simulink model "Pacejka_Tyre_Model"  (R2023b)
settings: Solver=VariableStepAuto  StartTime=0.0  StopTime=20  MinStep=1e-1  RelTol=1e-3
PostLoadFcn:
  | % loading model params:
  | load('pacajeka_model_param');
values from neighbouring files (symbols this model uses):
  a0 = 1.6    [pacajeka_init.m]    (also in pacajeka_model_param.mat)
  a1 = -34    [pacajeka_init.m]    (also in pacajeka_model_param.mat)
  a2 = 1250    [pacajeka_init.m]    (also in pacajeka_model_param.mat)
  a3 = 2320    [pacajeka_init.m]    (also in pacajeka_model_param.mat)
  a4 = 12.8    [pacajeka_init.m]    (also in pacajeka_model_param.mat)
  a5 = 0    [pacajeka_init.m]    (also in pacajeka_model_param.mat)
  a6 = -0.0053    [pacajeka_init.m]    (also in pacajeka_model_param.mat)
  a7 = 0.1925    [pacajeka_init.m]    (also in pacajeka_model_param.mat)
  a8 = 0    [pacajeka_init.m]    (also in pacajeka_model_param.mat)
  b0 = 1.55    [pacajeka_init.m]    (also in pacajeka_model_param.mat)
  b1 = 0    [pacajeka_init.m]    (also in pacajeka_model_param.mat)
  b2 = 1000    [pacajeka_init.m]    (also in pacajeka_model_param.mat)
  b3 = 60    [pacajeka_init.m]    (also in pacajeka_model_param.mat)
  b4 = 300    [pacajeka_init.m]    (also in pacajeka_model_param.mat)
  b5 = 0.17    [pacajeka_init.m]    (also in pacajeka_model_param.mat)
  b6 = 0    [pacajeka_init.m]    (also in pacajeka_model_param.mat)
  b7 = 0    [pacajeka_init.m]    (also in pacajeka_model_param.mat)
  b8 = 0.2    [pacajeka_init.m]    (also in pacajeka_model_param.mat)
settings Model: Creator=Milosh Yokich  LastModifiedBy=Milosh Yokich
settings DataIOCC: ExternalInput=[t_sim, Fz_sim, slip_sim, mu_sim, alpha_sim]  LoadExternalInput=on

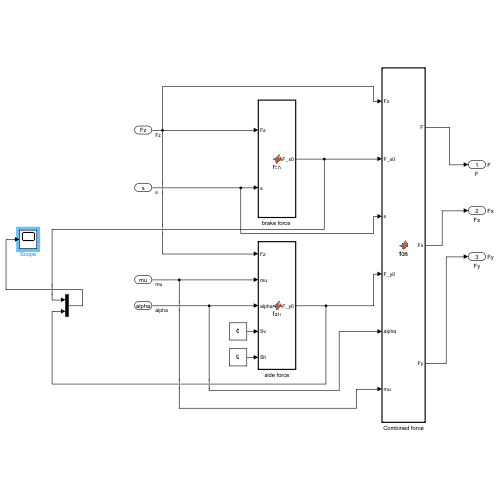
[thumbnail: Simulink's stored preview of the top-level diagram]
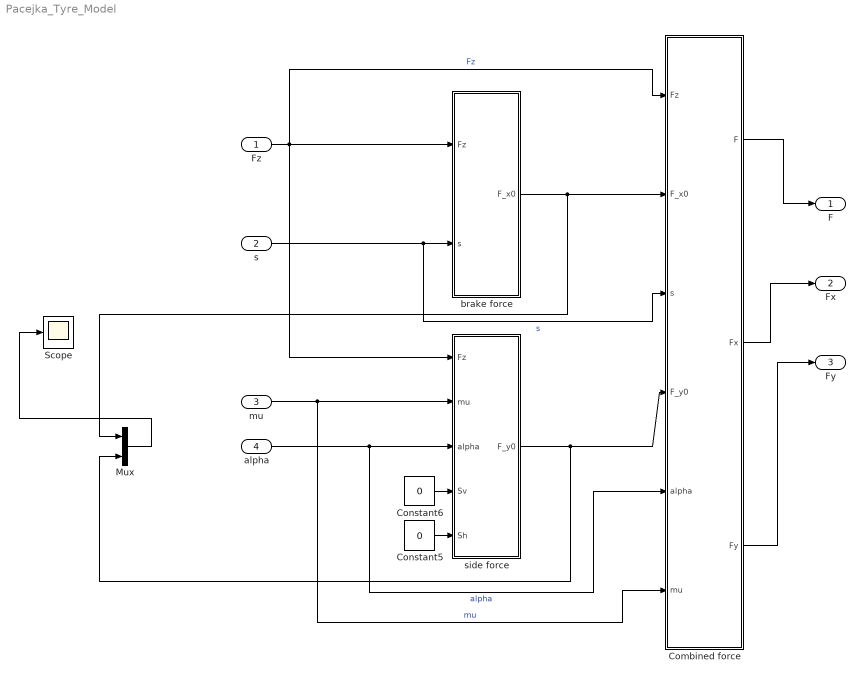
== system Pacejka_Tyre_Model ==
  Fz : Inport
  s : Inport  Port=2
  mu : Inport  Port=3
  alpha : Inport  Port=4
  Combined force : MATLAB Function  TreatAsAtomicUnit=on
  Constant5 : Constant  Value=0
  Constant6 : Constant  Value=0
  Mux : Mux  Inputs=2
  Scope : Scope
  "brake force " : MATLAB Function  TreatAsAtomicUnit=on
  side force : MATLAB Function  TreatAsAtomicUnit=on
  F : Outport  SignalName=F
  Fx : Outport  Port=2  SignalName=Fx
  Fy : Outport  Port=3  SignalName=Fy
  wires:
  Fz/1 -> "brake force "/1(Fz), Combined force/1(Fz), side force/1(Fz)  "Fz"
  Constant6/1 -> side force/4(Sv)
  Constant5/1 -> side force/5(Sh)
  "brake force "/1(F_x0) -> Mux/1, Combined force/2(F_x0)
  side force/1(F_y0) -> Mux/2, Combined force/4(F_y0)
  s/1 -> Combined force/3(s), "brake force "/2(s)  "s"
  mu/1 -> Combined force/6(mu), side force/2(mu)  "mu"
  alpha/1 -> Combined force/5(alpha), side force/3(alpha)  "alpha"
  Combined force/1(F) -> F/1
  Combined force/2(Fx) -> Fx/1
  Combined force/3(Fy) -> Fy/1
  Mux/1 -> Scope/1

== matlab function Pacejka_Tyre_Model/side force ==
  data: Fz input; mu input; alpha input; Sv input; Sh input; F_y0 output; a0 parameter; a1 parameter; a2 parameter; a3 parameter; a4 parameter; a6 parameter; a7 parameter; a5 parameter; a8 parameter
function F_y0 = fcn(Fz, mu, alpha, Sv, Sh, a0, a1, a2, a3, a4, a6, ...
    a7, a5, a8)
persistent C D B E

% init persistent variables: 
if isempty(C)
    C = a0;
    D = mu*(a1*Fz^2 + a2*Fz);
    B = (a3*sin(2*atan(Fz/a4)))/C/D;
    E = a6*Fz +a7;

end
X = alpha + Sh;
F_y0 = (D*sin(C*atan(B*((1-E)*X + E/B*atan(B*X)))) + Sv);

== matlab function Pacejka_Tyre_Model/brake force  ==
  data: Fz input; s input; F_x0 output; b0 parameter; b1 parameter; b2 parameter; b3 parameter; b4 parameter; b6 parameter; b7 parameter; b5 parameter; b8 parameter
function F_x0 = fcn(Fz, s, b0, b1, b2, b3, b4, b6, b7, b5, b8)
persistent C D B E

% init persistent variables: 
if isempty(C)
    C = b0;
    D = (b1*Fz^2 + b2*Fz);
    B = (b3*Fz^2 + b4*Fz)/(C*D*exp(b5*Fz));
    E = b6*Fz^2 + b7*Fz + b8;

end
X = s;
F_x0 = -(D*sin(C*atan(B*((1-E)*X + E/B*atan(B*X)))));

== matlab function Pacejka_Tyre_Model/Combined force ==
  data: Fz input; F_x0 input; F output; s input; F_y0 input; alpha input; Fx output; Fy output; mu input; b0 parameter; b1 parameter; b2 parameter; b3 parameter; b4 parameter; b6 parameter; b7 parameter; b5 parameter; a0 parameter; b8 parameter; a1 parameter; a2 parameter; a3 parameter; a4 parameter; a6 parameter; a7 parameter; a5 parameter; a8 parameter
function [F, Fx, Fy] = fcn(Fz, F_x0, s, F_y0, alpha, mu, b0, b1, b2, b3, ...
b4, b6, b7, b5, a0, b8, a1, a2, a3, a4, a6, a7, a5, a8)

persistent Cs Ds Bs Es Cl Dl Bl El C_s C_a
% init persistent variables, side force: 
if isempty(Cs)
    Cs = a0;
    Ds = mu*(a1*Fz^2 + a2*Fz);
    Bs = (a3*sin(2*atan(Fz/a4)))/Cs/Ds;
    Es = a6*Fz +a7;

    phi_s = (1-Es)*100 + Es/Bs*atan(Bs*100);
    Ps = Ds*sin(Cs*atan(Bs*phi_s));
    C_a = Bs*Cs*180/pi/Ps*mu*Fz;
end

% init persistent variables, longitudal force: 
if isempty(Cl)
    Cl = b0;
    Dl = (b1*Fz^2 + b2*Fz);
    Bl = (b3*Fz^2 + b4*Fz)/(Cl*Dl*exp(b5*Fz));
    El = b6*Fz^2 + b7*Fz + b8;

    phi_l = (1-El)*100 + El/Bl*atan(Bl*100);
    Pl = Dl*sin(Cl*atan(Bl*phi_l));
    C_s = Bl*Cl/Pl*mu*Fz*100;
end
% normalization of s
s = s/100;
alpha_rad = alpha/180*pi;

beta = atan2(sin(alpha_rad), s);

Fx = F_x0*F_y0/sqrt(s^2*F_y0^2 + F_x0^2*tan(alpha_rad)^2)*s;
if isnan(Fx)
    Fx = F_x0;
end
Fx = F_x0*abs(cos(beta));

Fy =  F_x0*F_y0/sqrt(s^2*F_y0^2 + F_x0^2*tan(alpha_rad)^2)*tan(alpha_rad);
if isnan(Fy)
    Fy = F_y0;
end
Fy = F_y0*abs(sin(beta));

F =  F_x0*cos(beta)^2 + F_y0*sin(beta)^2;
